simulink model "novel_wave"  (R2019a)
settings: Solver=VariableStepAuto  StartTime=0.0  StopTime=50  MaxStep=0.5  RelTol=1e-3
undefined symbols (not defined in the file or in its folder): magnitude
libraries: eeGeneralControl x1
settings Model: Creator=huic  LastModifiedBy=huic
settings DebuggingCC: AlgebraicLoopMsg=none

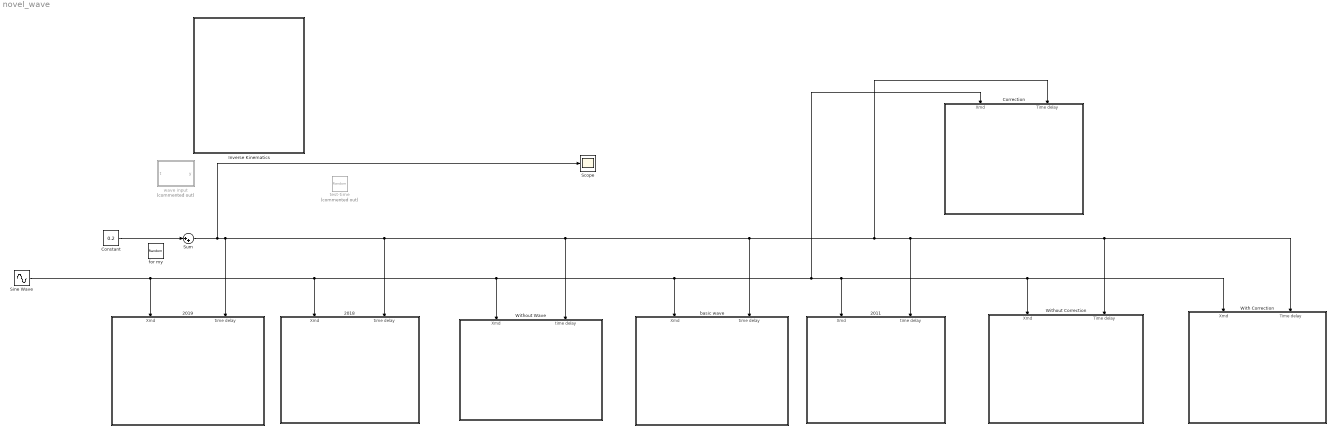
== system novel_wave ==
  2011 : Subsystem
  2018 : Subsystem
  2019 : Subsystem
  Constant : Constant  Value=0.2
  Correction : Subsystem
  Inverse Kinematics : Subsystem
  Scope : Scope
  Sine Wave : Sin  SampleTime=0
  Sum : Sum  Inputs=|++
  With Correction : Subsystem
  Without Correction : Subsystem
  Without Wave : Subsystem
  basic wave : Subsystem
  for my : RandomNumber  Mean=0.002  Variance=0.004  SampleTime=0.5
  test-time : RandomNumber  Commented=on  Mean=0.05  Variance=0.05  SampleTime=0.1
  wave input : MATLAB Function  Commented=on  TreatAsAtomicUnit=on
  wires:
  Constant/1 -> Sum/1
  Sum/1 -> Correction/2(Time delay), With Correction/2(Time delay), Without Correction/2(Time delay), 2011/2(time delay), basic wave/2(time delay), Without Wave/2(time delay), 2018/2(time delay), 2019/2(time delay), Scope/1
  Sine Wave/1 -> Correction/1(Xmd), With Correction/1(Xmd), Without Correction/1(Xmd), 2011/1(Xmd), basic wave/1(Xmd), Without Wave/1(Xmd), 2018/1(Xmd), 2019/1(Xmd)

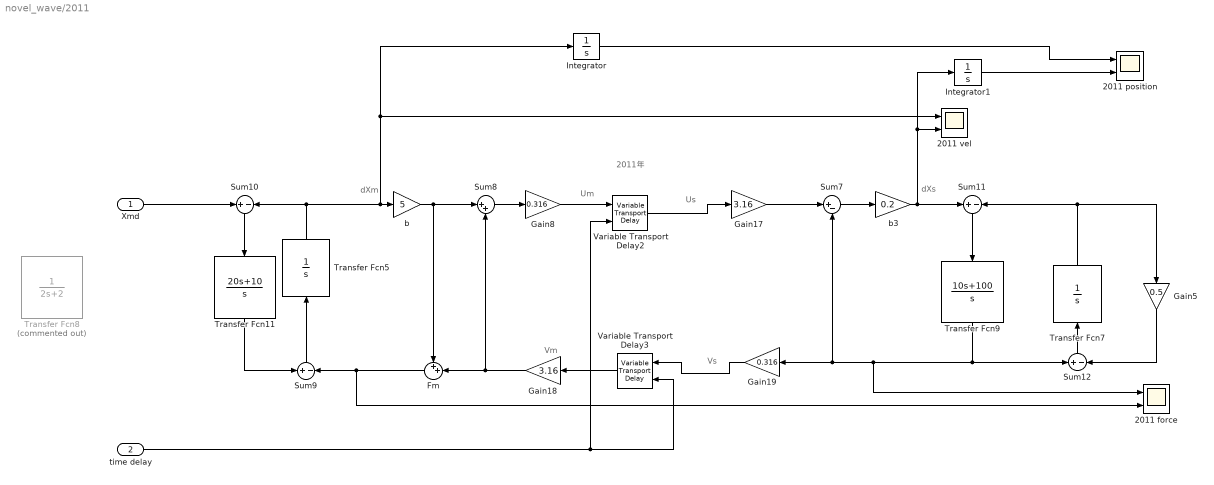
== system novel_wave/2011 ==
  note: 2011年
  note: Vm
  note: Us
  note: Um
  note: Vs
  note: dXm
  note: dXs
  Xmd : Inport
  time delay : Inport  Port=2
  2011 force : Scope  NumInputPorts=2
  2011 position : Scope  NumInputPorts=2
  2011 vel : Scope  NumInputPorts=2
  Fm : Sum  Inputs=++|
  Gain17 : Gain  Gain=3.16
  Gain18 : Gain  Gain=3.16
  Gain19 : Gain  Gain=0.316
  Gain5 : Gain  Gain=0.5
  Gain8 : Gain  Gain=0.316
  Integrator : Integrator
  Integrator1 : Integrator
  Sum{9..12} (4 alike) : Sum  Inputs=+|-
  Sum7 : Sum  Inputs=|+-
  Sum8 : Sum  Inputs=|++
  Transfer Fcn11 : TransferFcn  Numerator=[20 10]  Denominator=[1 0]
  Transfer Fcn5 : TransferFcn  Denominator=[1 0]
  Transfer Fcn7 : TransferFcn  Denominator=[1 0]
  Transfer Fcn8 : TransferFcn  Commented=on  Denominator=[2 2]
  Transfer Fcn9 : TransferFcn  Numerator=[10 100]  Denominator=[1 0]
  Variable Transport Delay2 : VariableTransportDelay  MaximumDelay=10  MaximumPoints=8069  ZeroDelay=on
  Variable Transport Delay3 : VariableTransportDelay  MaximumDelay=10  MaximumPoints=8069  ZeroDelay=on
  b : Gain  Gain=5
  b3 : Gain  Gain=0.2
  wires:
  Variable Transport Delay3/1 -> Gain18/1
  Variable Transport Delay2/1 -> Gain17/1
  Xmd/1 -> Sum10/1
  Fm/1 -> 2011 force/2, Sum9/2
  Gain5/1 -> Sum12/2
  Transfer Fcn9/1 -> 2011 force/1, Gain19/1, Sum7/2, Sum12/1
  Sum11/1 -> Transfer Fcn9/1
  b/1 -> Sum8/1, Fm/1
  Sum7/1 -> b3/1
  Gain19/1 -> Variable Transport Delay3/1
  Gain8/1 -> Variable Transport Delay2/1
  Gain17/1 -> Sum7/1
  Sum8/1 -> Gain8/1
  Transfer Fcn5/1 -> Integrator/1, 2011 vel/1, b/1, Sum10/2
  Gain18/1 -> Fm/2, Sum8/2
  Transfer Fcn7/1 -> Gain5/1, Sum11/2
  Sum9/1 -> Transfer Fcn5/1
  b3/1 -> Sum11/1, Integrator1/1, 2011 vel/2
  Sum12/1 -> Transfer Fcn7/1
  time delay/1 -> Variable Transport Delay2/2, Variable Transport Delay3/2
  Sum10/1 -> Transfer Fcn11/1
  Transfer Fcn11/1 -> Sum9/1
  Integrator/1 -> 2011 position/1
  Integrator1/1 -> 2011 position/2

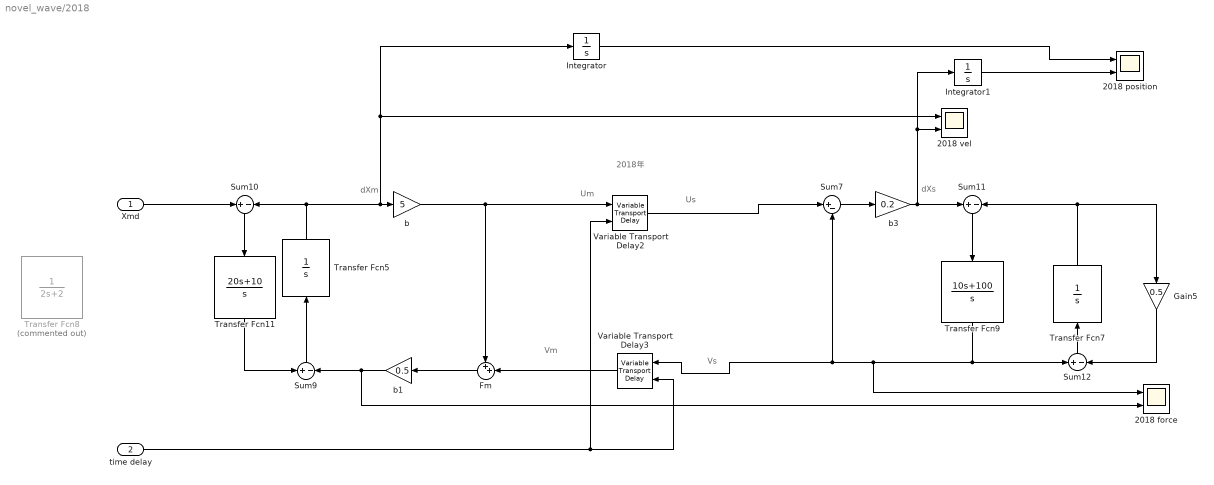
== system novel_wave/2018 ==
  note: 2018年
  note: Vm
  note: Us
  note: Um
  note: Vs
  note: dXm
  note: dXs
  Xmd : Inport
  time delay : Inport  Port=2
  2018 force : Scope  NumInputPorts=2
  2018 position : Scope  NumInputPorts=2
  2018 vel : Scope  NumInputPorts=2
  Fm : Sum  Inputs=++|
  Gain5 : Gain  Gain=0.5
  Integrator : Integrator
  Integrator1 : Integrator
  Sum{9..12} (4 alike) : Sum  Inputs=+|-
  Sum7 : Sum  Inputs=|+-
  Transfer Fcn11 : TransferFcn  Numerator=[20 10]  Denominator=[1 0]
  Transfer Fcn5 : TransferFcn  Denominator=[1 0]
  Transfer Fcn7 : TransferFcn  Denominator=[1 0]
  Transfer Fcn8 : TransferFcn  Commented=on  Denominator=[2 2]
  Transfer Fcn9 : TransferFcn  Numerator=[10 100]  Denominator=[1 0]
  Variable Transport Delay2 : VariableTransportDelay  MaximumDelay=10  MaximumPoints=8069  ZeroDelay=on
  Variable Transport Delay3 : VariableTransportDelay  MaximumDelay=10  MaximumPoints=8069  ZeroDelay=on
  b : Gain  Gain=5
  b1 : Gain  Gain=0.5
  b3 : Gain  Gain=0.2
  wires:
  Xmd/1 -> Sum10/1
  Gain5/1 -> Sum12/2
  Sum11/1 -> Transfer Fcn9/1
  Sum7/1 -> b3/1
  Transfer Fcn9/1 -> 2018 force/1, Variable Transport Delay3/1, Sum7/2, Sum12/1
  b/1 -> Variable Transport Delay2/1, Fm/1
  Variable Transport Delay2/1 -> Sum7/1
  Transfer Fcn5/1 -> Integrator/1, 2018 vel/1, b/1, Sum10/2
  Variable Transport Delay3/1 -> Fm/2
  Transfer Fcn7/1 -> Gain5/1, Sum11/2
  Sum9/1 -> Transfer Fcn5/1
  b3/1 -> Sum11/1, Integrator1/1, 2018 vel/2
  Sum12/1 -> Transfer Fcn7/1
  time delay/1 -> Variable Transport Delay2/2, Variable Transport Delay3/2
  Sum10/1 -> Transfer Fcn11/1
  Transfer Fcn11/1 -> Sum9/1
  Integrator/1 -> 2018 position/1
  Integrator1/1 -> 2018 position/2
  b1/1 -> 2018 force/2, Sum9/2
  Fm/1 -> b1/1

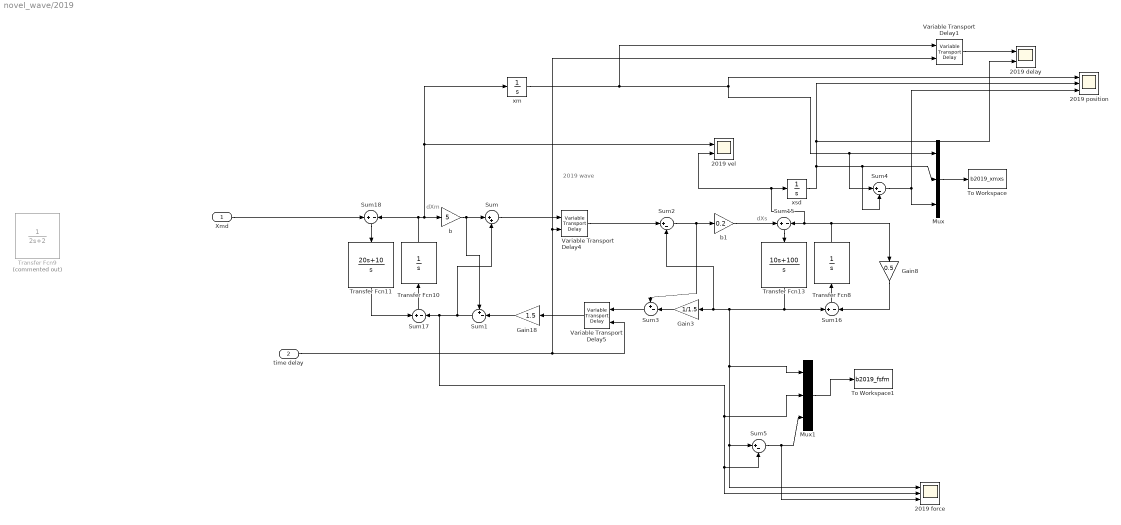
== system novel_wave/2019 ==
  note: 2019 wave
  note: dXm
  note: dXs
  Xmd : Inport
  time delay : Inport  Port=2
  2019 delay : Scope  NumInputPorts=2
  2019 force : Scope  NumInputPorts=3
  2019 position : Scope  NumInputPorts=3
  2019 vel : Scope  NumInputPorts=2
  Gain18 : Gain  Gain=1.5
  Gain3 : Gain  Gain=1/1.5
  Gain8 : Gain  Gain=0.5
  Mux : Mux  Inputs=3
  Mux1 : Mux  Inputs=3
  Sum : Sum  Inputs=|++
  Sum1 : Sum  Inputs=+-|
  Sum{15..18} (4 alike) : Sum  Inputs=+|-
  Sum2 : Sum  Inputs=|+-
  Sum3 : Sum  Inputs=+-|
  Sum4 : Sum  Inputs=|+-
  Sum5 : Sum  Inputs=|+-
  To Workspace : ToWorkspace  VariableName=b2019_xmxs  SaveFormat=Structure With Time  SampleTime=-1
  To Workspace1 : ToWorkspace  VariableName=b2019_fsfm  SaveFormat=Structure With Time  SampleTime=-1
  Transfer Fcn10 : TransferFcn  Denominator=[1 0]
  Transfer Fcn11 : TransferFcn  Numerator=[20 10]  Denominator=[1 0]
  Transfer Fcn13 : TransferFcn  Numerator=[10 100]  Denominator=[1 0]
  Transfer Fcn8 : TransferFcn  Denominator=[1 0]
  Transfer Fcn9 : TransferFcn  Commented=on  Denominator=[2 2]
  Variable Transport Delay1 : VariableTransportDelay  MaximumDelay=10  MaximumPoints=8069  ZeroDelay=on
  Variable Transport Delay4 : VariableTransportDelay  MaximumDelay=10  MaximumPoints=8069  ZeroDelay=on
  Variable Transport Delay5 : VariableTransportDelay  MaximumDelay=10  MaximumPoints=8069  ZeroDelay=on
  b : Gain  Gain=5
  b1 : Gain  Gain=0.2
  xm : Integrator
  xsd : Integrator
  wires:
  Gain8/1 -> Sum16/2
  Sum16/1 -> Transfer Fcn8/1
  Sum/1 -> Variable Transport Delay4/1
  Sum17/1 -> Transfer Fcn10/1
  Gain18/1 -> Sum1/2
  Sum2/1 -> b1/1, Sum3/1
  Transfer Fcn10/1 -> Sum18/2, xm/1, 2019 vel/1, b/1
  Xmd/1 -> Sum18/1
  b/1 -> Sum1/1, Sum/1
  Transfer Fcn13/1 -> Sum5/1, 2019 force/1, Mux1/1, Gain3/1, Sum2/2, Sum16/1
  Transfer Fcn8/1 -> Gain8/1, 2019 vel/2, xsd/1, Sum15/2
  b1/1 -> Sum15/1
  Sum15/1 -> Transfer Fcn13/1
  Variable Transport Delay5/1 -> Gain18/1
  Variable Transport Delay4/1 -> Sum2/1
  time delay/1 -> Variable Transport Delay5/2, Variable Transport Delay1/2, Variable Transport Delay4/2
  xsd/1 -> 2019 delay/2, 2019 position/2, Sum4/2, Mux/2
  Sum18/1 -> Transfer Fcn11/1
  Transfer Fcn11/1 -> Sum17/1
  Mux/1 -> To Workspace/1
  Mux1/1 -> To Workspace1/1
  xm/1 -> Variable Transport Delay1/1, Sum4/1, Mux/1, 2019 position/1
  Variable Transport Delay1/1 -> 2019 delay/1
  Sum1/1 -> Sum/2, 2019 force/2, Sum5/2, Mux1/2, Sum17/2
  Sum3/1 -> Variable Transport Delay5/1
  Gain3/1 -> Sum3/2
  Sum4/1 -> 2019 position/3, Mux/3
  Sum5/1 -> 2019 force/3, Mux1/3

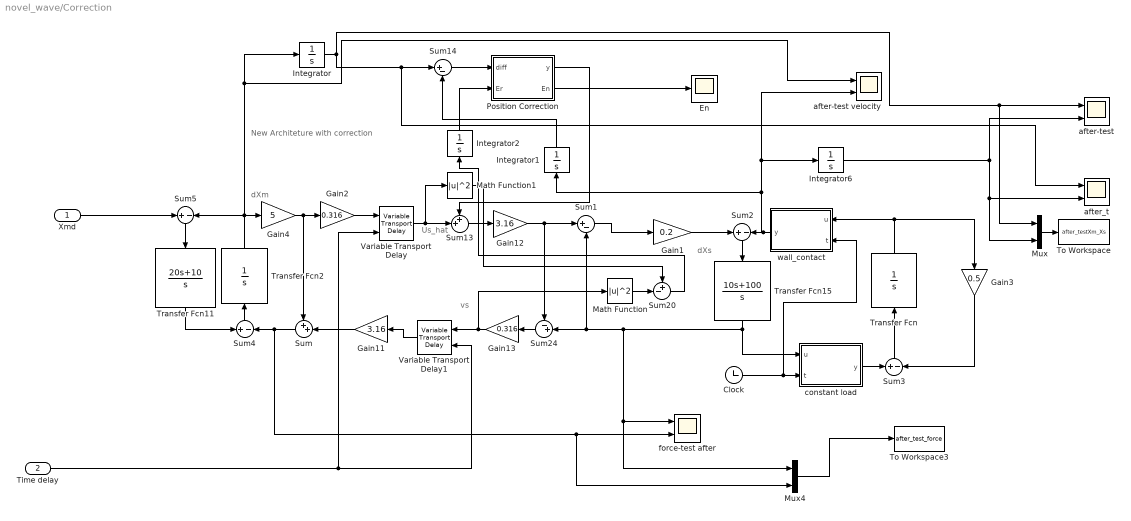
== system novel_wave/Correction ==
  note: vs
  note: dXm
  note: dXs
  note: New Architeture with correction
  note: Us_hat
  Xmd : Inport
  Time delay : Inport  Port=2
  Clock : Clock
  En : Scope
  Gain1 : Gain  Gain=0.2
  Gain11 : Gain  Gain=3.16
  Gain12 : Gain  Gain=3.16
  Gain13 : Gain  Gain=0.316
  Gain2 : Gain  Gain=0.316
  Gain3 : Gain  Gain=0.5
  Gain4 : Gain  Gain=5
  Integrator{,1..2,6} (4 alike) : Integrator
  Math Function : Math  Operator=magnitude^2  SaturateOnIntegerOverflow=on
  Math Function1 : Math  Operator=magnitude^2  SaturateOnIntegerOverflow=on
  Mux : Mux  Inputs=2
  Mux4 : Mux  Inputs=2
  "Position Correction " : MATLAB Function  TreatAsAtomicUnit=on
  Sum : Sum  Inputs=++|
  Sum1 : Sum  Inputs=|+-
  Sum13 : Sum  Inputs=++|
  Sum14 : Sum  Inputs=|+-
  Sum{2..5} (4 alike) : Sum  Inputs=+|-
  Sum20 : Sum  Inputs=+-|
  Sum24 : Sum  Inputs=-+|
  To Workspace : ToWorkspace  VariableName=after_testXm_Xs  SaveFormat=Structure With Time  SampleTime=-1
  To Workspace3 : ToWorkspace  VariableName=after_test_force  SaveFormat=Structure With Time  SampleTime=-1
  Transfer Fcn : TransferFcn  Denominator=[1 0]
  Transfer Fcn11 : TransferFcn  Numerator=[20 10]  Denominator=[1 0]
  Transfer Fcn15 : TransferFcn  Numerator=[10 100]  Denominator=[1 0]
  Transfer Fcn2 : TransferFcn  Denominator=[1 0]
  Variable Transport Delay : VariableTransportDelay  MaximumDelay=10  MaximumPoints=8069  ZeroDelay=on
  Variable Transport Delay1 : VariableTransportDelay  MaximumDelay=10  MaximumPoints=8069  ZeroDelay=on
  after-test : Scope  NumInputPorts=2
  after-test velocity : Scope  NumInputPorts=2
  after_t : Scope  NumInputPorts=2
  constant load : MATLAB Function  TreatAsAtomicUnit=on
  force-test after : Scope  NumInputPorts=2
  wall_contact : MATLAB Function  TreatAsAtomicUnit=on
  wires:
  Sum2/1 -> Transfer Fcn15/1
  Integrator2/1 -> "Position Correction "/2(Er)
  Math Function/1 -> Sum20/2
  Sum4/1 -> Transfer Fcn2/1
  constant load/1(y) -> Sum3/1
  Mux/1 -> To Workspace/1
  Gain2/1 -> Variable Transport Delay/1
  Transfer Fcn15/1 -> Mux4/1, force-test after/1, Sum24/2, Sum1/2, constant load/1(u)
  Transfer Fcn2/1 -> Gain4/1, after-test velocity/1, Integrator/1, Sum5/2
  "Position Correction "/2(En) -> En/1
  Transfer Fcn11/1 -> Sum4/1
  Integrator1/1 -> Sum14/2
  Sum5/1 -> Transfer Fcn11/1
  Gain3/1 -> Sum3/2
  Gain4/1 -> Gain2/1, Sum/1
  Sum20/1 -> Integrator2/1
  Integrator6/1 -> after-test/2, after_t/2, Mux/2
  Clock/1 -> wall_contact/2(t), constant load/2(t)
  Math Function1/1 -> Sum20/1
  Sum13/1 -> Gain12/1
  Transfer Fcn/1 -> wall_contact/1(u), Gain3/1
  Sum3/1 -> Transfer Fcn/1
  Sum14/1 -> "Position Correction "/1(diff)
  Gain1/1 -> Sum2/1
  Mux4/1 -> To Workspace3/1
  wall_contact/1(y) -> Integrator6/1, after-test velocity/2, Integrator1/1, Sum2/2
  Gain12/1 -> Sum1/1, Sum24/1
  Variable Transport Delay1/1 -> Gain11/1
  Sum/1 -> Mux4/2, force-test after/2, Sum4/2
  Variable Transport Delay/1 -> Math Function1/1, Sum13/2
  Sum24/1 -> Gain13/1
  Gain13/1 -> Math Function/1, Variable Transport Delay1/1
  Gain11/1 -> Sum/2
  Sum1/1 -> Gain1/1
  Xmd/1 -> Sum5/1
  Time delay/1 -> Variable Transport Delay/2, Variable Transport Delay1/2
  "Position Correction "/1(y) -> Sum13/1
  Integrator/1 -> Sum14/1, after_t/1, Mux/1, after-test/1

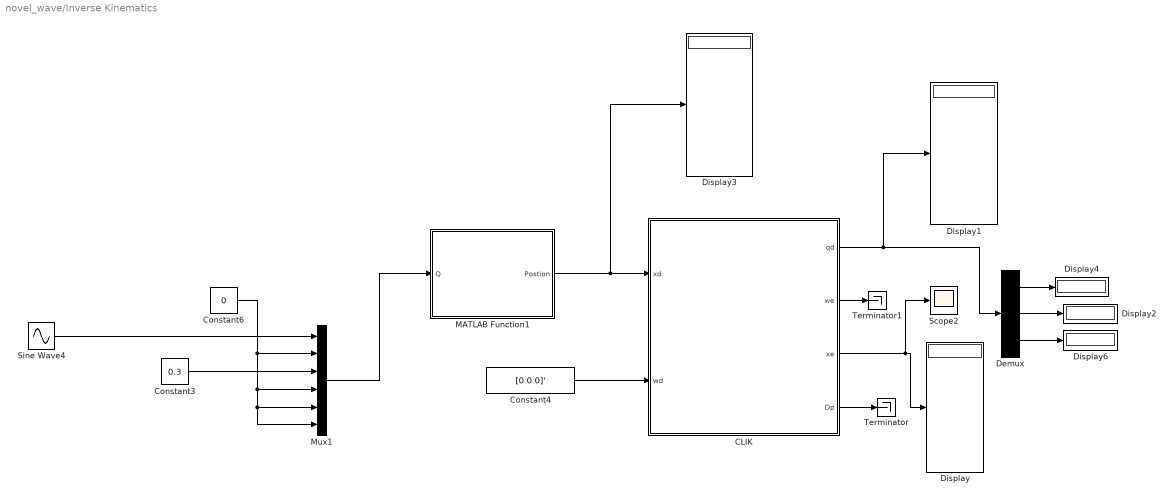
== system novel_wave/Inverse Kinematics ==
  CLIK : Subsystem
  Constant3 : Constant  Value=0.3
  Constant4 : Constant  Value=[0 0 0]'
  Constant6 : Constant  Value=0
  Demux : Demux  Outputs=3
  Display{,1..4,6} (6 alike) : Display
  MATLAB Function1 : MATLAB Function  TreatAsAtomicUnit=on
  Mux1 : Mux  Inputs=6
  Scope2 : Scope
  Sine Wave4 : Sin  Amplitude=-0.8  Frequency=0.5  SampleTime=0
  Terminator : Terminator
  Terminator1 : Terminator
  wires:
  CLIK/4(Dp) -> Terminator/1
  CLIK/3(xe) -> Scope2/1, Display/1
  Constant6/1 -> Mux1/6, Mux1/5, Mux1/4, Mux1/2
  Sine Wave4/1 -> Mux1/1
  CLIK/2(we) -> Terminator1/1
  Mux1/1 -> MATLAB Function1/1(Q)
  Demux/3 -> Display6/1
  CLIK/1(qd) -> Demux/1, Display1/1
  MATLAB Function1/1(Postion) -> Display3/1, CLIK/1(xd)
  Constant4/1 -> CLIK/2(wd)
  Constant3/1 -> Mux1/3
  Demux/1 -> Display4/1
  Demux/2 -> Display2/1

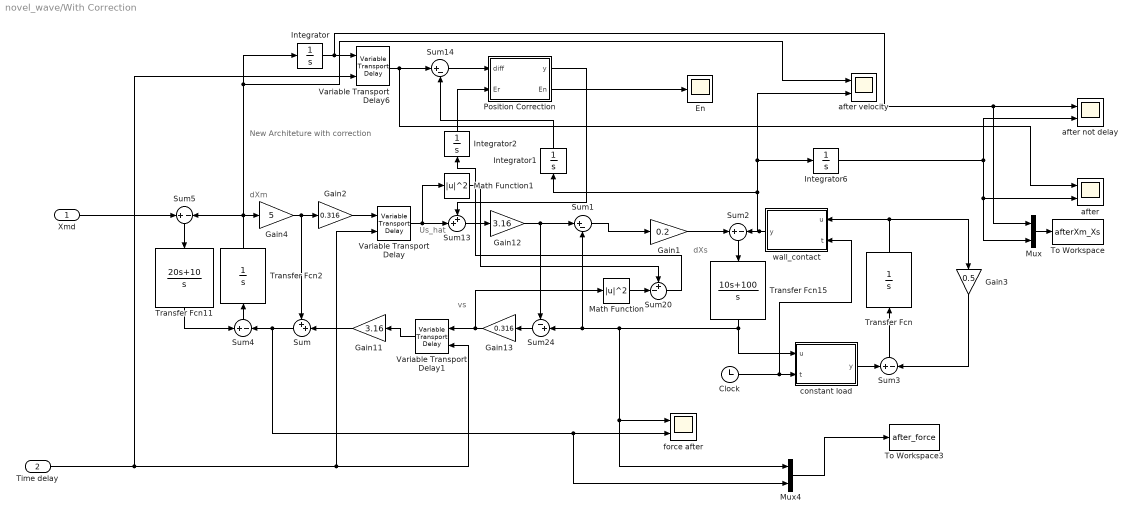
== system novel_wave/With Correction ==
  note: vs
  note: dXm
  note: dXs
  note: New Architeture with correction
  note: Us_hat
  Xmd : Inport
  Time delay : Inport  Port=2
  Clock : Clock
  En : Scope
  Gain1 : Gain  Gain=0.2
  Gain11 : Gain  Gain=3.16
  Gain12 : Gain  Gain=3.16
  Gain13 : Gain  Gain=0.316
  Gain2 : Gain  Gain=0.316
  Gain3 : Gain  Gain=0.5
  Gain4 : Gain  Gain=5
  Integrator{,1..2,6} (4 alike) : Integrator
  Math Function : Math  Operator=magnitude^2  SaturateOnIntegerOverflow=on
  Math Function1 : Math  Operator=magnitude^2  SaturateOnIntegerOverflow=on
  Mux : Mux  Inputs=2
  Mux4 : Mux  Inputs=2
  "Position Correction " : MATLAB Function  TreatAsAtomicUnit=on
  Sum : Sum  Inputs=++|
  Sum1 : Sum  Inputs=|+-
  Sum13 : Sum  Inputs=++|
  Sum14 : Sum  Inputs=|+-
  Sum{2..5} (4 alike) : Sum  Inputs=+|-
  Sum20 : Sum  Inputs=+-|
  Sum24 : Sum  Inputs=-+|
  To Workspace : ToWorkspace  VariableName=afterXm_Xs  SaveFormat=Structure With Time  SampleTime=-1
  To Workspace3 : ToWorkspace  VariableName=after_force  SaveFormat=Structure With Time  SampleTime=-1
  Transfer Fcn : TransferFcn  Denominator=[1 0]
  Transfer Fcn11 : TransferFcn  Numerator=[20 10]  Denominator=[1 0]
  Transfer Fcn15 : TransferFcn  Numerator=[10 100]  Denominator=[1 0]
  Transfer Fcn2 : TransferFcn  Denominator=[1 0]
  Variable Transport Delay : VariableTransportDelay  MaximumDelay=10  MaximumPoints=8069  ZeroDelay=on
  Variable Transport Delay1 : VariableTransportDelay  MaximumDelay=10  MaximumPoints=8069  ZeroDelay=on
  Variable Transport Delay6 : VariableTransportDelay  MaximumDelay=10  MaximumPoints=8069  ZeroDelay=on
  after : Scope  NumInputPorts=2
  after not delay : Scope  NumInputPorts=2
  after velocity : Scope  NumInputPorts=2
  constant load : MATLAB Function  TreatAsAtomicUnit=on
  force after : Scope  NumInputPorts=2
  wall_contact : MATLAB Function  TreatAsAtomicUnit=on
  wires:
  Sum2/1 -> Transfer Fcn15/1
  Integrator2/1 -> "Position Correction "/2(Er)
  Math Function/1 -> Sum20/2
  Sum4/1 -> Transfer Fcn2/1
  constant load/1(y) -> Sum3/1
  Mux/1 -> To Workspace/1
  Gain2/1 -> Variable Transport Delay/1
  Transfer Fcn15/1 -> Mux4/1, force after/1, Sum24/2, Sum1/2, constant load/1(u)
  Transfer Fcn2/1 -> Gain4/1, after velocity/1, Integrator/1, Sum5/2
  "Position Correction "/2(En) -> En/1
  Transfer Fcn11/1 -> Sum4/1
  Integrator1/1 -> Sum14/2
  Sum5/1 -> Transfer Fcn11/1
  Gain3/1 -> Sum3/2
  Gain4/1 -> Gain2/1, Sum/1
  Sum20/1 -> Integrator2/1
  Integrator6/1 -> after not delay/2, after/2, Mux/2
  Clock/1 -> wall_contact/2(t), constant load/2(t)
  Math Function1/1 -> Sum20/1
  Integrator/1 -> Mux/1, after not delay/1, Variable Transport Delay6/1
  Sum13/1 -> Gain12/1
  Transfer Fcn/1 -> wall_contact/1(u), Gain3/1
  Sum3/1 -> Transfer Fcn/1
  Sum14/1 -> "Position Correction "/1(diff)
  Gain1/1 -> Sum2/1
  Mux4/1 -> To Workspace3/1
  wall_contact/1(y) -> after velocity/2, Integrator6/1, Integrator1/1, Sum2/2
  Gain12/1 -> Sum1/1, Sum24/1
  Variable Transport Delay1/1 -> Gain11/1
  Sum/1 -> Mux4/2, force after/2, Sum4/2
  Variable Transport Delay/1 -> Math Function1/1, Sum13/2
  Sum24/1 -> Gain13/1
  Gain13/1 -> Math Function/1, Variable Transport Delay1/1
  Gain11/1 -> Sum/2
  Sum1/1 -> Gain1/1
  Xmd/1 -> Sum5/1
  Time delay/1 -> Variable Transport Delay/2, Variable Transport Delay1/2, Variable Transport Delay6/2
  "Position Correction "/1(y) -> Sum13/1
  Variable Transport Delay6/1 -> Sum14/1, after/1

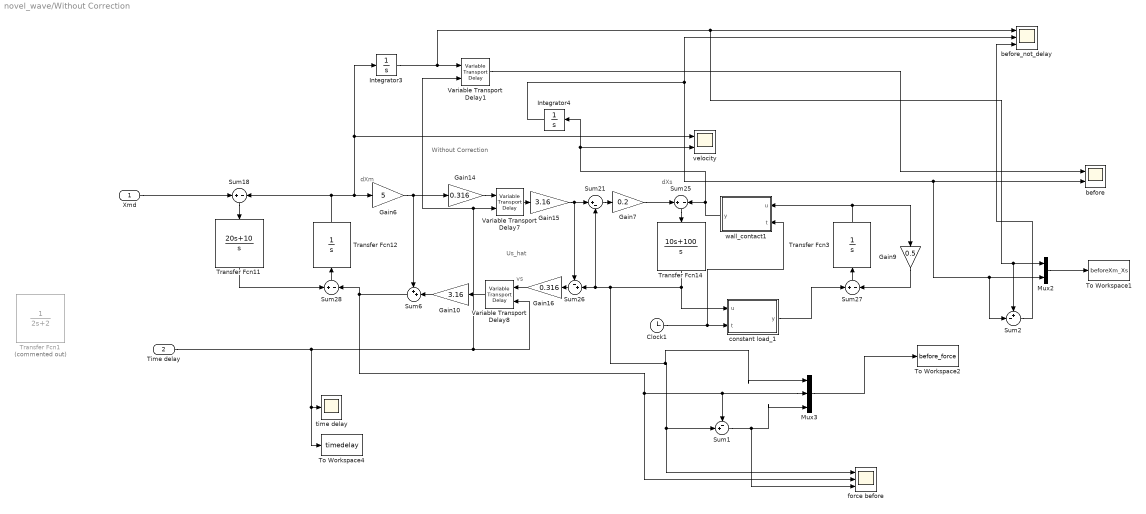
== system novel_wave/Without Correction ==
  note: vs
  note: Us_hat
  note: dXs
  note: dXm
  note: Without Correction
  Xmd : Inport
  Time delay : Inport  Port=2
  Clock1 : Clock
  Gain10 : Gain  Gain=3.16
  Gain14 : Gain  Gain=0.316
  Gain15 : Gain  Gain=3.16
  Gain16 : Gain  Gain=0.316
  Gain6 : Gain  Gain=5
  Gain7 : Gain  Gain=0.2
  Gain9 : Gain  Gain=0.5
  Integrator3 : Integrator
  Integrator4 : Integrator
  Mux2 : Mux  Inputs=2
  Mux3 : Mux  Inputs=3
  Sum1 : Sum  Inputs=-+|
  Sum{18,25,27..28} (4 alike) : Sum  Inputs=+|-
  Sum2 : Sum  Inputs=+-|
  Sum21 : Sum  Inputs=|+-
  Sum26 : Sum  Inputs=-+|
  Sum6 : Sum  Inputs=++|
  To Workspace1 : ToWorkspace  VariableName=beforeXm_Xs  SaveFormat=Structure With Time  SampleTime=-1
  To Workspace2 : ToWorkspace  VariableName=before_force  SaveFormat=Structure With Time  SampleTime=-1
  To Workspace4 : ToWorkspace  VariableName=timedelay  SaveFormat=Structure With Time  SampleTime=-1
  Transfer Fcn1 : TransferFcn  Commented=on  Denominator=[2 2]
  Transfer Fcn11 : TransferFcn  Numerator=[20 10]  Denominator=[1 0]
  Transfer Fcn12 : TransferFcn  Denominator=[1 0]
  Transfer Fcn14 : TransferFcn  Numerator=[10 100]  Denominator=[1 0]
  Transfer Fcn3 : TransferFcn  Denominator=[1 0]
  Variable Transport Delay1 : VariableTransportDelay  MaximumDelay=10  MaximumPoints=4068  ZeroDelay=on
  Variable Transport Delay7 : VariableTransportDelay  MaximumDelay=10  MaximumPoints=4068  ZeroDelay=on
  Variable Transport Delay8 : VariableTransportDelay  MaximumDelay=10  MaximumPoints=4068  ZeroDelay=on
  before : Scope  NumInputPorts=2
  before_not_delay : Scope  NumInputPorts=3
  constant load_1 : MATLAB Function  TreatAsAtomicUnit=on
  force before : Scope  NumInputPorts=3
  time delay : Scope
  velocity : Scope  NumInputPorts=2
  wall_contact1 : MATLAB Function  TreatAsAtomicUnit=on
  wires:
  Clock1/1 -> wall_contact1/2(t), constant load_1/2(t)
  Transfer Fcn3/1 -> wall_contact1/1(u), Gain9/1
  Transfer Fcn12/1 -> Sum18/2, velocity/1, Integrator3/1, Gain6/1
  Gain15/1 -> Sum21/1, Sum26/1
  Gain14/1 -> Variable Transport Delay7/1
  Gain7/1 -> Sum25/1
  Sum27/1 -> Transfer Fcn3/1
  Gain9/1 -> Sum27/2
  Mux3/1 -> To Workspace2/1
  Sum6/1 -> Sum28/2, Sum1/1, Mux3/2, force before/2
  wall_contact1/1(y) -> velocity/2, Integrator4/1, Sum25/2
  Mux2/1 -> To Workspace1/1
  Integrator4/1 -> before/2, Sum2/2, Mux2/2, before_not_delay/2
  Transfer Fcn14/1 -> Mux3/1, Sum1/2, force before/1, Sum26/2, Sum21/2, constant load_1/1(u)
  constant load_1/1(y) -> Sum27/1
  Sum28/1 -> Transfer Fcn12/1
  Gain6/1 -> Gain14/1, Sum6/1
  Gain10/1 -> Sum6/2
  Xmd/1 -> Sum18/1
  Variable Transport Delay7/1 -> Gain15/1
  Gain16/1 -> Variable Transport Delay8/1
  Sum21/1 -> Gain7/1
  Variable Transport Delay8/1 -> Gain10/1
  Sum26/1 -> Gain16/1
  Sum25/1 -> Transfer Fcn14/1
  Time delay/1 -> To Workspace4/1, time delay/1, Variable Transport Delay1/2, Variable Transport Delay7/2, Variable Transport Delay8/2
  Integrator3/1 -> Mux2/1, Sum2/1, before_not_delay/1, Variable Transport Delay1/1
  Variable Transport Delay1/1 -> before/1
  Sum18/1 -> Transfer Fcn11/1
  Transfer Fcn11/1 -> Sum28/1
  Sum1/1 -> force before/3, Mux3/3
  Sum2/1 -> before_not_delay/3

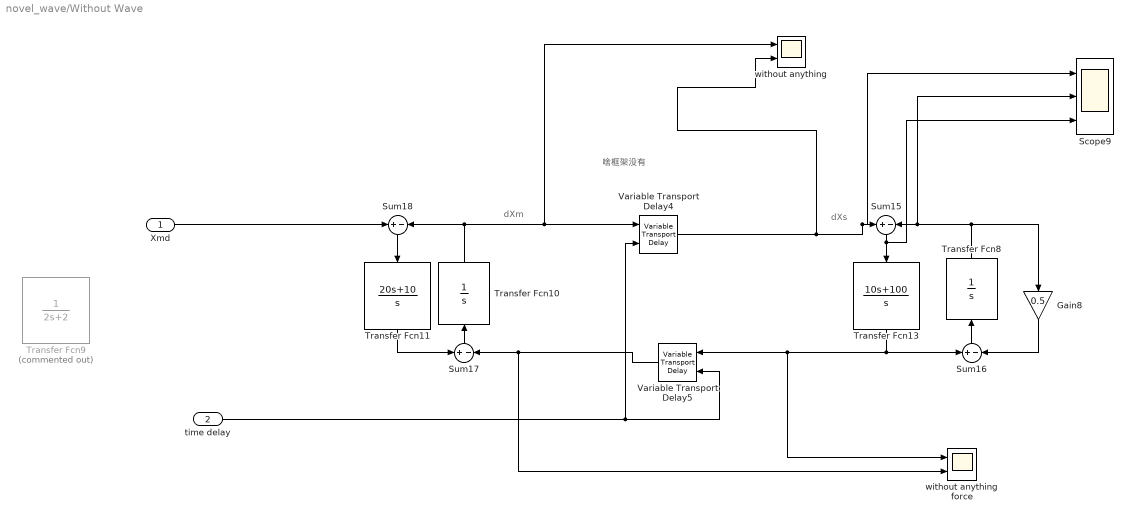
== system novel_wave/Without Wave ==
  note: 啥框架没有
  note: dXm
  note: dXs
  Xmd : Inport
  time delay : Inport  Port=2
  Gain8 : Gain  Gain=0.5
  Scope9 : Scope  NumInputPorts=3
  Sum{15..18} (4 alike) : Sum  Inputs=+|-
  Transfer Fcn10 : TransferFcn  Denominator=[1 0]
  Transfer Fcn11 : TransferFcn  Numerator=[20 10]  Denominator=[1 0]
  Transfer Fcn13 : TransferFcn  Numerator=[10 100]  Denominator=[1 0]
  Transfer Fcn8 : TransferFcn  Denominator=[1 0]
  Transfer Fcn9 : TransferFcn  Commented=on  Denominator=[2 2]
  Variable Transport Delay4 : VariableTransportDelay  MaximumDelay=10  MaximumPoints=8069  ZeroDelay=on
  Variable Transport Delay5 : VariableTransportDelay  MaximumDelay=10  MaximumPoints=8069  ZeroDelay=on
  without anything : Scope  NumInputPorts=2
  without anything force : Scope  NumInputPorts=2
  wires:
  Gain8/1 -> Sum16/2
  Transfer Fcn13/1 -> without anything force/1, Variable Transport Delay5/1, Sum16/1
  Variable Transport Delay5/1 -> without anything force/2, Sum17/2
  Transfer Fcn8/1 -> Gain8/1, Scope9/2, Sum15/2
  Sum15/1 -> Transfer Fcn13/1, Scope9/3
  Sum17/1 -> Transfer Fcn10/1
  Sum16/1 -> Transfer Fcn8/1
  time delay/1 -> Variable Transport Delay4/2, Variable Transport Delay5/2
  Transfer Fcn10/1 -> without anything/1, Variable Transport Delay4/1, Sum18/2
  Variable Transport Delay4/1 -> without anything/2, Scope9/1, Sum15/1
  Xmd/1 -> Sum18/1
  Sum18/1 -> Transfer Fcn11/1
  Transfer Fcn11/1 -> Sum17/1

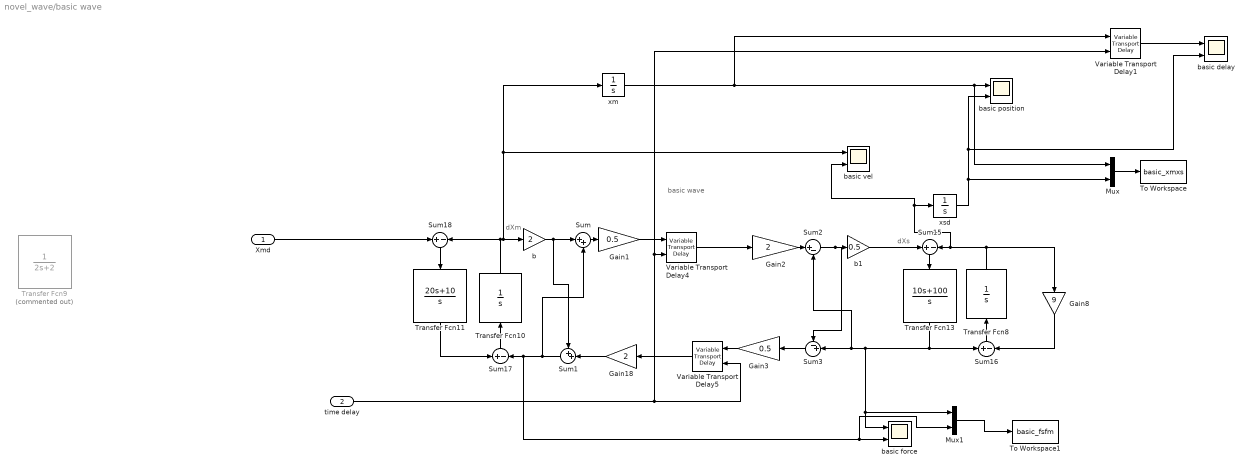
== system novel_wave/basic wave ==
  note: basic wave
  note: dXm
  note: dXs
  Xmd : Inport
  time delay : Inport  Port=2
  Gain1 : Gain  Gain=0.5
  Gain18 : Gain  Gain=2
  Gain2 : Gain  Gain=2
  Gain3 : Gain  Gain=0.5
  Gain8 : Gain  Gain=9
  Mux : Mux  Inputs=2
  Mux1 : Mux  Inputs=2
  Sum : Sum  Inputs=|++
  Sum1 : Sum  Inputs=++|
  Sum{15..18} (4 alike) : Sum  Inputs=+|-
  Sum2 : Sum  Inputs=|+-
  Sum3 : Sum  Inputs=-+|
  To Workspace : ToWorkspace  VariableName=basic_xmxs  SaveFormat=Structure With Time  SampleTime=-1
  To Workspace1 : ToWorkspace  VariableName=basic_fsfm  SaveFormat=Structure With Time  SampleTime=-1
  Transfer Fcn10 : TransferFcn  Denominator=[1 0]
  Transfer Fcn11 : TransferFcn  Numerator=[20 10]  Denominator=[1 0]
  Transfer Fcn13 : TransferFcn  Numerator=[10 100]  Denominator=[1 0]
  Transfer Fcn8 : TransferFcn  Denominator=[1 0]
  Transfer Fcn9 : TransferFcn  Commented=on  Denominator=[2 2]
  Variable Transport Delay1 : VariableTransportDelay  MaximumDelay=10  MaximumPoints=8069  ZeroDelay=on
  Variable Transport Delay4 : VariableTransportDelay  MaximumDelay=10  MaximumPoints=8069  ZeroDelay=on
  Variable Transport Delay5 : VariableTransportDelay  MaximumDelay=10  MaximumPoints=8069  ZeroDelay=on
  b : Gain  Gain=2
  b1 : Gain  Gain=0.5
  basic delay : Scope  NumInputPorts=2
  basic force : Scope  NumInputPorts=2
  basic position : Scope  NumInputPorts=2
  basic vel : Scope  NumInputPorts=2
  xm : Integrator
  xsd : Integrator
  wires:
  Gain8/1 -> Sum16/2
  Sum16/1 -> Transfer Fcn8/1
  Gain1/1 -> Variable Transport Delay4/1
  Sum17/1 -> Transfer Fcn10/1
  Gain18/1 -> Sum1/2
  Sum2/1 -> b1/1, Sum3/1
  Transfer Fcn10/1 -> b/1, xm/1, basic vel/1, Sum18/2
  Xmd/1 -> Sum18/1
  b/1 -> Sum1/1, Sum/1
  Transfer Fcn13/1 -> Mux1/1, basic force/1, Sum3/2, Sum2/2, Sum16/1
  Transfer Fcn8/1 -> Gain8/1, basic vel/2, xsd/1, Sum15/2
  Sum1/1 -> Sum/2, Mux1/2, basic force/2, Sum17/2
  b1/1 -> Sum15/1
  Sum15/1 -> Transfer Fcn13/1
  Sum/1 -> Gain1/1
  Variable Transport Delay5/1 -> Gain18/1
  Gain2/1 -> Sum2/1
  time delay/1 -> Variable Transport Delay5/2, Variable Transport Delay1/2, Variable Transport Delay4/2
  xsd/1 -> basic delay/2, basic position/2, Mux/2
  Sum18/1 -> Transfer Fcn11/1
  Transfer Fcn11/1 -> Sum17/1
  Mux/1 -> To Workspace/1
  Mux1/1 -> To Workspace1/1
  Variable Transport Delay4/1 -> Gain2/1
  xm/1 -> Variable Transport Delay1/1, basic position/1, Mux/1
  Variable Transport Delay1/1 -> basic delay/1
  Sum3/1 -> Gain3/1
  Gain3/1 -> Variable Transport Delay5/1

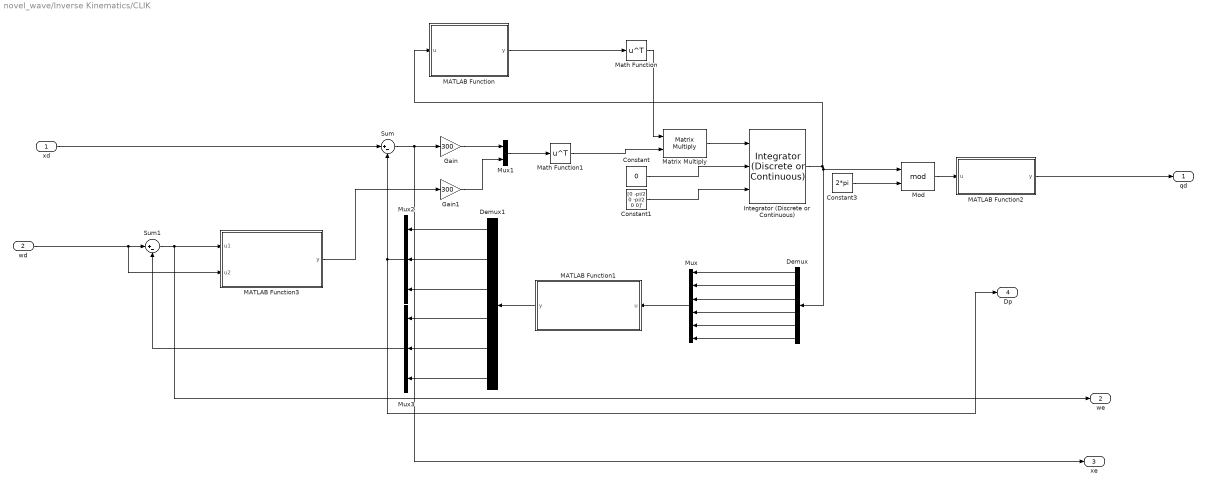
== system novel_wave/Inverse Kinematics/CLIK ==
  xd : Inport
  wd : Inport  Port=2
  Constant : Constant  Value=0
  Constant1 : Constant  Value=[0 -pi/2 0 -pi/2 0 0]'
  Constant3 : Constant  Value=2*pi
  Demux : Demux  Outputs=[1 1 1 1 1 1]
  Demux1 : Demux  Outputs=[1 1 1 1 1 1]
  Gain : Gain  Gain=300
  Gain1 : Gain  Gain=300
  Integrator (Discrete or Continuous) : eeGeneralControl/Integrator (Discrete or Continuous)  LabelModeActiveChoice=Continuous  ExternalReset=level  LimitType=Anti-windup  B=inf  A=-inf  Ts=0
      settings: SourceProductName=Simscape Electrical  SourceProductBaseCode=PS
  MATLAB Function : MATLAB Function  TreatAsAtomicUnit=on
  MATLAB Function1 : MATLAB Function  TreatAsAtomicUnit=on
  MATLAB Function2 : MATLAB Function  TreatAsAtomicUnit=on
  MATLAB Function3 : MATLAB Function  TreatAsAtomicUnit=on
  Math Function : Math  Operator=transpose  SaturateOnIntegerOverflow=on
  Math Function1 : Math  Operator=transpose  SaturateOnIntegerOverflow=on
  Matrix Multiply : Product  Multiplication=Matrix(*)
  Mod : Math  Operator=mod  SaturateOnIntegerOverflow=on
  Mux : Mux  Inputs=[1 1 1 1 1 1]
  Mux1 : Mux  Inputs=2
  Mux2 : Mux  Inputs=[1 1 1]
  Mux3 : Mux  Inputs=[1 1 1]
  Sum : Sum  Inputs=|+-
  Sum1 : Sum  Inputs=|+-
  qd : Outport
  we : Outport  Port=2
  xe : Outport  Port=3
  Dp : Outport  Port=4
  wires:
  Demux/2 -> Mux/2
  Gain/1 -> Mux1/1
  Integrator (Discrete or Continuous)/1 -> MATLAB Function/1(u), Demux/1, Mod/1
  Math Function/1 -> Matrix Multiply/1
  Demux/5 -> Mux/5
  Mux/1 -> MATLAB Function1/1(u)
  MATLAB Function2/1(y) -> qd/1
  Mux1/1 -> Math Function1/1
  Demux/4 -> Mux/4
  Demux1/5 -> Mux3/2
  MATLAB Function3/1(y) -> Gain1/1
  Demux/6 -> Mux/6
  wd/1 -> MATLAB Function3/2(u2), Sum1/1
  Demux/1 -> Mux/1
  Demux/3 -> Mux/3
  Matrix Multiply/1 -> Integrator (Discrete or Continuous)/1
  Sum/1 -> xe/1, Gain/1
  Mux3/1 -> Sum1/2
  Constant3/1 -> Mod/2
  Mux2/1 -> Dp/1, Sum/2
  Demux1/4 -> Mux3/1
  Mod/1 -> MATLAB Function2/1(u)
  Demux1/1 -> Mux2/1
  Demux1/2 -> Mux2/2
  Gain1/1 -> Mux1/2
  MATLAB Function1/1(y) -> Demux1/1
  Math Function1/1 -> Matrix Multiply/2
  Demux1/3 -> Mux2/3
  Sum1/1 -> we/1, MATLAB Function3/1(u1)
  Constant1/1 -> Integrator (Discrete or Continuous)/3
  Demux1/6 -> Mux3/3
  xd/1 -> Sum/1
  Constant/1 -> Integrator (Discrete or Continuous)/2
  MATLAB Function/1(y) -> Math Function/1

== matlab function novel_wave/With Correction/constant load ==
  data: u input; y output; t input
function y = constantload(u,t)
% if t > 20
%     u = u + 0.05;
% end
y = u;

== matlab function novel_wave/With Correction/Position Correction  ==
  data: diff input; y output; Er input; En output
function [y,En] = fcn(diff,Er)
%1-exp(-0.5*Er)
%1/(1+exp(-0.5*Er))
% 
% if Er > 0.7 
%     Er = 0;
% end
y=5*(1-exp(-0.5*Er))*sqrt(5/2)/2*diff;
En=1/(1-exp(-0.5*Er));

== matlab function novel_wave/Without Correction/constant load_1 ==
  data: u input; y output; t input
function y = constantload(u,t)
% if t > 20
%     u = u + 0.05;
% end
y = u;

== matlab function novel_wave/With Correction/wall_contact ==
  data: u input; y output; t input
function y = wall_contact(u,t)
% if t > 20 && t <40 
%     u = 0;
% end
y = u;

== matlab function novel_wave/Without Correction/wall_contact1 ==
  data: u input; y output; t input
function y = wall_contact(u,t)
% if t > 20 && t <40 
%     u = 0;
% end
y = u;

== matlab function novel_wave/Inverse Kinematics/MATLAB Function1 ==
  data: Q input; Postion output
function Postion = TouchX_to_Gluon(Q)
d4=0.13335;d6=0.03;a2=0.13335;
q1=Q(1);q2=Q(2);q3=Q(3);q4=Q(4);q5=Q(5);q6=Q(6);
T01=[cos(q1) -sin(q1) 0 0;sin(q1) cos(q1) 0 0;0 0 1 0;0 0 0 1];
T12=[cos(q2) -sin(q2) 0 0;0 0 -1 0;sin(q2) cos(q2) 0 0;0 0 0 1];
T23=[cos(q3) -sin(q3) 0 a2;sin(q3) cos(q3) 0 0;0 0 1 0;0 0 0 1];
T34=[cos(q4) -sin(q4) 0 0;0 0 -1 -d4;sin(q4) cos(q4) 0 0;0 0 0 1];
T45=[cos(q5) -sin(q5) 0 0;0 0 -1 0;sin(q5) cos(q5) 0 0;0 0 0 1];
T56=[cos(q6) -sin(q6) 0 0;0 0 1 d6;-sin(q6) -cos(q6) 0 0;0 0 0 1];

T06=T01*T12*T23*T34*T45*T56;
%进行映射转换
 Xg = 2.4*T06(1,4)-0.26;
 Yg = 1.6*T06(2,4)-0.05;
 Zg = 1.4*T06(3,4)+0.11;
 %对映射后的X、Y空间做约束
 %将Xg限制在【-0.05,0.05】之外
 if Xg > -0.05 && Xg <= 0 && Yg > -0.05 && Yg < 0.05
    Xg = -0.05;
 elseif Xg < 0.05 && Xg >=0  && Yg > -0.05 && Yg < 0.05
        Xg = 0.05;
 end
         
%进行映射后的笛卡尔空间位置
P=[Xg;Yg;Zg];
% pose=tform2eul(T06);
Postion = P;
% Pose=pose';

== matlab function novel_wave/Inverse Kinematics/CLIK/MATLAB Function ==
  data: u input; y output
function y = getjacob(u)
%标准型雅可比矩阵求解
a2=-0.2035;a3=-0.17442;d1=0.1205;d4=0.08009;
d5=0.08009;d6=0.04436;
q=u;
%求运动学正解
T01 = [cos(q(1)) 0 sin(q(1)) 0;sin(q(1)) 0 -cos(q(1)) 0;0 1 0 d1;0 0 0 1];
T12 = [cos(q(2)) -sin(q(2)) 0 a2*cos(q(2));sin(q(2)) cos(q(2)) 0 a2*sin(q(2));0 0 1 0;0 0 0 1];
T23 = [cos(q(3)) -sin(q(3)) 0 a3*cos(q(3));sin(q(3)) cos(q(3)) 0 a3*sin(q(3));0 0 1 0;0 0 0 1];
T34 = [cos(q(4)) 0 sin(q(4)) 0;sin(q(4)) 0 -cos(q(4)) 0;0 1 0 d4;0 0 0 1];
T45 = [cos(q(5)) 0 -sin(q(5))  0;sin(q(5)) 0 cos(q(5)) 0;0 -1 0 d5;0 0 0 1];
T56 = [cos(q(6)) -sin(q(6)) 0 0;sin(q(6)) cos(q(6)) 0 0;0 0 1 d6;0 0 0 1];

k = [0; 0; 1];

%初始赋值
Jv = zeros(3, 6);
Jw = zeros(3, 6);
%获取每个关节原点与基座标的变换矩阵T01,T02...T06
% T{6}=zeros(4);
T=cell(6,1);
T{1}=T01;
T{2}=T{1}*T12;
T{3}=T{2}*T23;
T{4}=T{3}*T34;
T{5}=T{4}*T45;
T{6}=T{5}*T56;

%进行矢量积求解
for i = 1: 6
   if i == 1
       R = eye(3);
       p_im = T{6}(1: 3, 4);
   else
       R = T{i-1}(1: 3, 1: 3);
       p_im = T{6}(1: 3, 4) - T{i-1}(1: 3, 4);
   end
   
   zi_1 = R * k;
   Jv(:, i) = cross(zi_1, p_im);
   Jw(:, i) = zi_1;
end

% 组合
J = [Jv; Jw];
y=J;

== matlab function novel_wave/Inverse Kinematics/CLIK/MATLAB Function1 ==
  data: u input; y output
function y = getpose(u)
a2=-0.2035;a3=-0.17442;d1=0.1205;d4=0.08009;
d5=0.08009;d6=0.04436;
q1=u(1);
q2=u(2);
q3=u(3);
q4=u(4);
q5=u(5);
q6=u(6);
%求运动学正解
T01 = [cos(q1) 0 sin(q1) 0;sin(q1) 0 -cos(q1) 0;0 1 0 d1;0 0 0 1];
T12 = [cos(q2) -sin(q2) 0 a2*cos(q2);sin(q2) cos(q2) 0 a2*sin(q2);0 0 1 0;0 0 0 1];
T23 = [cos(q3) -sin(q3) 0 a3*cos(q3);sin(q3) cos(q3) 0 a3*sin(q3);0 0 1 0;0 0 0 1];
T34 = [cos(q4) 0 sin(q4) 0;sin(q4) 0 -cos(q4) 0;0 1 0 d4;0 0 0 1];
T45 = [cos(q5) 0 -sin(q5)  0;sin(q5) 0 cos(q5) 0;0 -1 0 d5;0 0 0 1];
T56 = [cos(q6) -sin(q6) 0 0;sin(q6) cos(q6) 0 0;0 0 1 d6;0 0 0 1];
T06 = T01*T12*T23*T34*T45*T56;

y1=T06(1:3,4);
y2=tform2eul(T06);
y=[y1;y2'];

== matlab function novel_wave/Inverse Kinematics/CLIK/MATLAB Function2 ==
  data: u input; y output
function y = Joints_angle_Handle(u)
for i=1:5
    if(u(i) > pi)
        u(i) = u(i)-2*pi;
    elseif(u(i) < -pi)
        u(i) = u(i)+2*pi;
    end
end

y = u;

== matlab function novel_wave/Inverse Kinematics/CLIK/MATLAB Function3 ==
  data: u1 input; y output; u2 input
function y = anglevelocity(u1,u2)
%u2为当前的欧拉角
%u1为欧拉角的变化量
tform=[cos(u2(2))*cos(u2(3)) -sin(u2(3)) 0;cos(u2(2))*sin(u2(3)) cos(u2(3)) 0;-sin(u2(2)) 0 1];
y=zeros(1,3);
dwxyz=tform*[u1(3);u1(2);u1(1)];
y(1)=dwxyz(1);
y(2)=dwxyz(2);
y(3)=dwxyz(3);

== matlab function novel_wave/wave input ==
  data: t input; y output
function y = wave_input(t)

if t < 10
    t = 0.2;
elseif t>=10 && t <20
    t = 0;
elseif t >= 20 && t < 30
    t = -0.2;
elseif t >= 30 && t < 40 
    t = 0;
elseif t >= 40 && t <= 50
    t = 0.2;
end
y=t;

== matlab function novel_wave/Correction/Position Correction  ==
  data: diff input; y output; Er input; En output
function [y,En] = fcn(diff,Er)
%1-exp(-0.5*Er)
%1/(1+exp(-0.5*Er))
y=5*(1-exp(-0.5*Er))*sqrt(5/2)/2*diff;
En=1/(1-exp(-0.5*Er));

== matlab function novel_wave/Correction/constant load ==
  data: u input; y output; t input
function y = constantload(u,t)
% if t > 20
%     u = u + 0.05;
% end
y = u;

== matlab function novel_wave/Correction/wall_contact ==
  data: u input; y output; t input
function y = wall_contact(u,t)
% if t > 20 && t <40 
%     u = 0;
% end
y = u;
